simulink library "oneTetCtrllr_cl"  (R2018b)
settings: Solver=VariableStepAuto  StartTime=0.0  StopTime=10.0  RelTol=1e-3
values from neighbouring files (symbols this model uses):
  ctrl = CTR.oneThrCtlr    [oneThrCtrl_ts.m]
libraries: filteredPIDController_ul x3
settings Model: Creator=asiddiq2  LastModifiedBy=asiddiq2

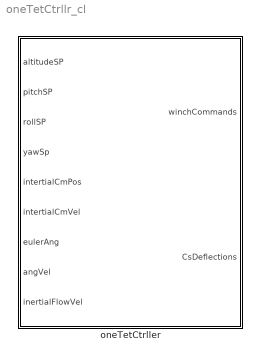
== system oneTetCtrllr_cl ==
  oneTetCtrller : Subsystem

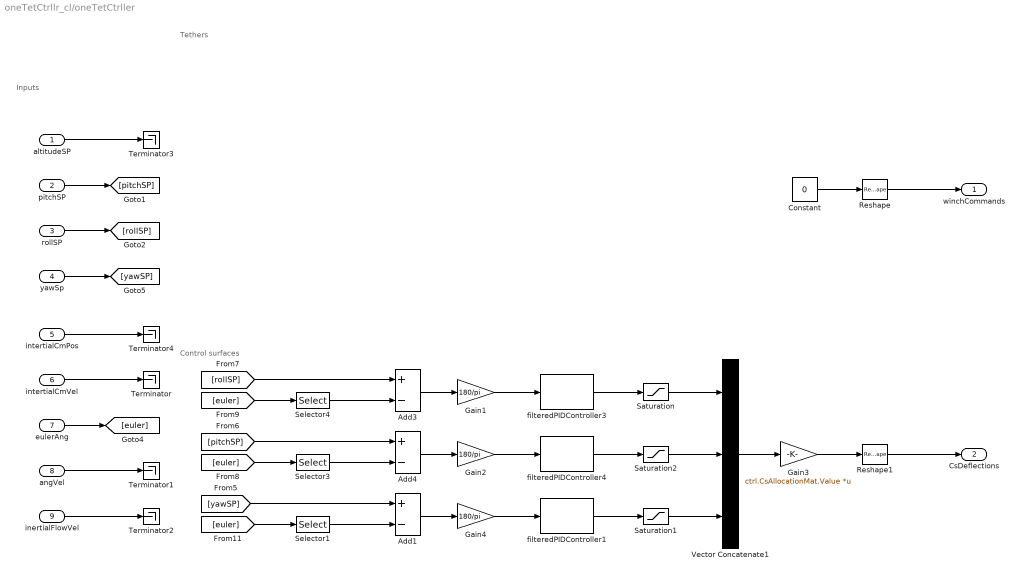
== system oneTetCtrllr_cl/oneTetCtrller ==
  note: Control surfaces
  note: Tethers
  note: Inputs
  altitudeSP : Inport
  pitchSP : Inport  Port=2
  rollSP : Inport  Port=3
  yawSp : Inport  Port=4
  intertialCmPos : Inport  Port=5
  intertialCmVel : Inport  Port=6
  eulerAng : Inport  Port=7
  angVel : Inport  Port=8
  inertialFlowVel : Inport  Port=9
  Add1 : Sum  Inputs=+-
  Add3 : Sum  Inputs=+-
  Add4 : Sum  Inputs=+-
  Constant : Constant  Value=0
  Gain1 : Gain  Gain=180/pi
  Gain2 : Gain  Gain=180/pi
  Gain3 : Gain  Gain=ctrl.CsAllocationMat.Value  Multiplication=Matrix(K*u)
  Gain4 : Gain  Gain=180/pi
  Reshape : Reshape  OutputDimensionality=Row vector (2-D)
  Reshape1 : Reshape  OutputDimensionality=Column vector (2-D)
  Saturation : Saturate  UpperLimit=ctrl.aileronMaxDef.Value  LowerLimit=-ctrl.aileronMaxDef.Value
  Saturation1 : Saturate  UpperLimit=ctrl.rudderMaxDef.Value  LowerLimit=-ctrl.rudderMaxDef.Value
  Saturation2 : Saturate  UpperLimit=ctrl.elevatorMaxDef.Value  LowerLimit=-ctrl.elevatorMaxDef.Value
  Selector1 : Selector  NumberOfDimensions=2  InputPortWidth=3  IndexOptions=Index vector (dialog),Index vector (dialog)  Indices=3,1  OutputSizes=1,1
  Selector3 : Selector  NumberOfDimensions=2  InputPortWidth=3  IndexOptions=Index vector (dialog),Index vector (dialog)  Indices=2,1  OutputSizes=1,1
  Selector4 : Selector  NumberOfDimensions=2  InputPortWidth=3  IndexOptions=Index vector (dialog),Index vector (dialog)  Indices=1,1  OutputSizes=1,1
  Terminator{,1..4} (5 alike) : Terminator
  Vector Concatenate1 : Concatenate  NumInputs=3
  filteredPIDController1 : filteredPIDController_ul/filteredPIDController  kp=ctrl.rudderKp.Value  ki=ctrl.rudderKi.Value  kd=ctrl.rudderKd.Value  Value=ctrl.rudderTau.Value
  filteredPIDController3 : filteredPIDController_ul/filteredPIDController  kp=ctrl.aileronKp.Value  ki=ctrl.aileronKi.Value  kd=ctrl.aileronKd.Value  Value=ctrl.aileronTau.Value
  filteredPIDController4 : filteredPIDController_ul/filteredPIDController  kp=ctrl.elevatorKp.Value  ki=ctrl.elevatorKi.Value  kd=ctrl.elevatorKd.Value  Value=ctrl.elevatorTau.Value
  winchCommands : Outport
  CsDeflections : Outport  Port=2
  wires:
  filteredPIDController3/1 -> Saturation/1
  Add3/1 -> Gain1/1
  Add4/1 -> Gain2/1
  [rollSP] -> Add3/1
  eulerAng/1 -> [euler]
  angVel/1 -> Terminator1/1
  Vector Concatenate1/1 -> Gain3/1
  altitudeSP/1 -> Terminator3/1
  filteredPIDController4/1 -> Saturation2/1
  intertialCmVel/1 -> Terminator/1
  Gain2/1 -> filteredPIDController4/1
  Selector1/1 -> Add1/2
  inertialFlowVel/1 -> Terminator2/1
  intertialCmPos/1 -> Terminator4/1
  [yawSP] -> Add1/1
  [euler] -> Selector4/1
  Selector4/1 -> Add3/2
  rollSP/1 -> [rollSP]
  filteredPIDController1/1 -> Saturation1/1
  Gain3/1 -> Reshape1/1
  Selector3/1 -> Add4/2
  Add1/1 -> Gain4/1
  [pitchSP] -> Add4/1
  Reshape1/1 -> CsDeflections/1
  [euler] -> Selector3/1
  Gain1/1 -> filteredPIDController3/1
  Reshape/1 -> winchCommands/1
  Gain4/1 -> filteredPIDController1/1
  Saturation/1 -> Vector Concatenate1/1
  Constant/1 -> Reshape/1
  yawSp/1 -> [yawSP]
  Saturation1/1 -> Vector Concatenate1/3
  Saturation2/1 -> Vector Concatenate1/2
  [euler] -> Selector1/1
  pitchSP/1 -> [pitchSP]
